simulink model "model"  (R2014a)
(part 6 of 6)

  bus4 : powerlib/Measurements/Load Flow Bus  LConnTagsString=a  ID=bus4  Vbase=10000  Vref=1  Vangle=0  VLF=1  angleLF=0
      settings: AttributesFormatString=|
      | %<ID>
      | %<Vbase>V
      | %<VLF>pu
      | %<angleLF>deg.
      | %<Name>
  bus40 : powerlib/Measurements/Load Flow Bus  LConnTagsString=a  ID=bus40  Vbase=10000  Vref=1  Vangle=0  VLF=1  angleLF=0
      settings: AttributesFormatString=|
      | %<ID>
      | %<Vbase>V
      | %<VLF>pu
      | %<angleLF>deg.
      | %<Name>
  bus41 : powerlib/Measurements/Load Flow Bus  LConnTagsString=a  ID=bus41  Vbase=10000  Vref=1  Vangle=0  VLF=1  angleLF=0
      settings: AttributesFormatString=|
      | %<ID>
      | %<Vbase>V
      | %<VLF>pu
      | %<angleLF>deg.
      | %<Name>
  bus42 : powerlib/Measurements/Load Flow Bus  LConnTagsString=a  ID=bus42  Vbase=10000  Vref=1  Vangle=0  VLF=1  angleLF=0
      settings: AttributesFormatString=|
      | %<ID>
      | %<Vbase>V
      | %<VLF>pu
      | %<angleLF>deg.
      | %<Name>
  bus43 : powerlib/Measurements/Load Flow Bus  LConnTagsString=a  ID=bus43  Vbase=10000  Vref=1  Vangle=0  VLF=1  angleLF=0
      settings: AttributesFormatString=|
      | %<ID>
      | %<Vbase>V
      | %<VLF>pu
      | %<angleLF>deg.
      | %<Name>
  bus44 : powerlib/Measurements/Load Flow Bus  LConnTagsString=a  ID=bus44  Vbase=10000  Vref=1  Vangle=0  VLF=1  angleLF=0
      settings: AttributesFormatString=|
      | %<ID>
      | %<Vbase>V
      | %<VLF>pu
      | %<angleLF>deg.
      | %<Name>
  bus45 : powerlib/Measurements/Load Flow Bus  LConnTagsString=a  ID=bus45  Vbase=10000  Vref=1  Vangle=0  VLF=1  angleLF=0
      settings: AttributesFormatString=|
      | %<ID>
      | %<Vbase>V
      | %<VLF>pu
      | %<angleLF>deg.
      | %<Name>
  bus46 : powerlib/Measurements/Load Flow Bus  LConnTagsString=a  ID=bus46  Vbase=10000  Vref=1  Vangle=0  VLF=1  angleLF=0
      settings: AttributesFormatString=|
      | %<ID>
      | %<Vbase>V
      | %<VLF>pu
      | %<angleLF>deg.
      | %<Name>
  bus47 : powerlib/Measurements/Load Flow Bus  LConnTagsString=a  ID=bus47  Vbase=10000  Vref=1  Vangle=0  VLF=1  angleLF=0
      settings: AttributesFormatString=|
      | %<ID>
      | %<Vbase>V
      | %<VLF>pu
      | %<angleLF>deg.
      | %<Name>
  bus48 : powerlib/Measurements/Load Flow Bus  LConnTagsString=a  ID=bus48  Vbase=10000  Vref=1  Vangle=0  VLF=1  angleLF=0
      settings: AttributesFormatString=|
      | %<ID>
      | %<Vbase>V
      | %<VLF>pu
      | %<angleLF>deg.
      | %<Name>
  bus49 : powerlib/Measurements/Load Flow Bus  LConnTagsString=a  ID=bus49  Vbase=10000  Vref=1  Vangle=0  VLF=1  angleLF=0
      settings: AttributesFormatString=|
      | %<ID>
      | %<Vbase>V
      | %<VLF>pu
      | %<angleLF>deg.
      | %<Name>
  bus5 : powerlib/Measurements/Load Flow Bus  LConnTagsString=a  ID=bus5  Vbase=10000  Vref=1  Vangle=0  VLF=1  angleLF=0
      settings: AttributesFormatString=|
      | %<ID>
      | %<Vbase>V
      | %<VLF>pu
      | %<angleLF>deg.
      | %<Name>
  bus50 : powerlib/Measurements/Load Flow Bus  LConnTagsString=a  ID=bus50  Vbase=10000  Vref=1  Vangle=0  VLF=1  angleLF=0
      settings: AttributesFormatString=|
      | %<ID>
      | %<Vbase>V
      | %<VLF>pu
      | %<angleLF>deg.
      | %<Name>
  bus51 : powerlib/Measurements/Load Flow Bus  LConnTagsString=a  ID=bus51  Vbase=10000  Vref=1  Vangle=0  VLF=1  angleLF=0
      settings: AttributesFormatString=|
      | %<ID>
      | %<Vbase>V
      | %<VLF>pu
      | %<angleLF>deg.
      | %<Name>
  bus52 : powerlib/Measurements/Load Flow Bus  LConnTagsString=a  ID=bus52  Vbase=10000  Vref=1  Vangle=0  VLF=1  angleLF=0
      settings: AttributesFormatString=|
      | %<ID>
      | %<Vbase>V
      | %<VLF>pu
      | %<angleLF>deg.
      | %<Name>
  bus53 : powerlib/Measurements/Load Flow Bus  LConnTagsString=a  ID=bus53  Vbase=10000  Vref=1  Vangle=0  VLF=1  angleLF=0
      settings: AttributesFormatString=|
      | %<ID>
      | %<Vbase>V
      | %<VLF>pu
      | %<angleLF>deg.
      | %<Name>
  bus54 : powerlib/Measurements/Load Flow Bus  LConnTagsString=a  ID=bus54  Vbase=10000  Vref=1  Vangle=0  VLF=1  angleLF=0
      settings: AttributesFormatString=|
      | %<ID>
      | %<Vbase>V
      | %<VLF>pu
      | %<angleLF>deg.
      | %<Name>
  bus55 : powerlib/Measurements/Load Flow Bus  LConnTagsString=a  ID=bus55  Vbase=10000  Vref=1  Vangle=0  VLF=1  angleLF=0
      settings: AttributesFormatString=|
      | %<ID>
      | %<Vbase>V
      | %<VLF>pu
      | %<angleLF>deg.
      | %<Name>
  bus56 : powerlib/Measurements/Load Flow Bus  LConnTagsString=a  ID=bus56  Vbase=10000  Vref=1  Vangle=0  VLF=1  angleLF=0
      settings: AttributesFormatString=|
      | %<ID>
      | %<Vbase>V
      | %<VLF>pu
      | %<angleLF>deg.
      | %<Name>
  bus57 : powerlib/Measurements/Load Flow Bus  LConnTagsString=a  ID=bus57  Vbase=10000  Vref=1  Vangle=0  VLF=1  angleLF=0
      settings: AttributesFormatString=|
      | %<ID>
      | %<Vbase>V
      | %<VLF>pu
      | %<angleLF>deg.
      | %<Name>
  bus58 : powerlib/Measurements/Load Flow Bus  LConnTagsString=a  ID=bus58  Vbase=10000  Vref=1  Vangle=0  VLF=1  angleLF=0
      settings: AttributesFormatString=|
      | %<ID>
      | %<Vbase>V
      | %<VLF>pu
      | %<angleLF>deg.
      | %<Name>
  bus59 : powerlib/Measurements/Load Flow Bus  LConnTagsString=a  ID=bus59  Vbase=10000  Vref=1  Vangle=0  VLF=1  angleLF=0
      settings: AttributesFormatString=|
      | %<ID>
      | %<Vbase>V
      | %<VLF>pu
      | %<angleLF>deg.
      | %<Name>
  bus6 : powerlib/Measurements/Load Flow Bus  LConnTagsString=a  ID=bus6  Vbase=10000  Vref=1  Vangle=0  VLF=1  angleLF=0
      settings: AttributesFormatString=|
      | %<ID>
      | %<Vbase>V
      | %<VLF>pu
      | %<angleLF>deg.
      | %<Name>
  bus60 : powerlib/Measurements/Load Flow Bus  LConnTagsString=a  ID=bus60  Vbase=10000  Vref=1  Vangle=0  VLF=1  angleLF=0
      settings: AttributesFormatString=|
      | %<ID>
      | %<Vbase>V
      | %<VLF>pu
      | %<angleLF>deg.
      | %<Name>
  bus61 : powerlib/Measurements/Load Flow Bus  LConnTagsString=a  ID=bus61  Vbase=10000  Vref=1  Vangle=0  VLF=1  angleLF=0
      settings: AttributesFormatString=|
      | %<ID>
      | %<Vbase>V
      | %<VLF>pu
      | %<angleLF>deg.
      | %<Name>
  bus62 : powerlib/Measurements/Load Flow Bus  LConnTagsString=a  ID=bus62  Vbase=10000  Vref=1  Vangle=0  VLF=1  angleLF=0
      settings: AttributesFormatString=|
      | %<ID>
      | %<Vbase>V
      | %<VLF>pu
      | %<angleLF>deg.
      | %<Name>
  bus63 : powerlib/Measurements/Load Flow Bus  LConnTagsString=a  ID=bus63  Vbase=10000  Vref=1  Vangle=0  VLF=1  angleLF=0
      settings: AttributesFormatString=|
      | %<ID>
      | %<Vbase>V
      | %<VLF>pu
      | %<angleLF>deg.
      | %<Name>
  bus64 : powerlib/Measurements/Load Flow Bus  LConnTagsString=a  ID=bus64  Vbase=10000  Vref=1  Vangle=0  VLF=1  angleLF=0
      settings: AttributesFormatString=|
      | %<ID>
      | %<Vbase>V
      | %<VLF>pu
      | %<angleLF>deg.
      | %<Name>
  bus65 : powerlib/Measurements/Load Flow Bus  LConnTagsString=a  ID=bus65  Vbase=10000  Vref=1  Vangle=0  VLF=1  angleLF=0
      settings: AttributesFormatString=|
      | %<ID>
      | %<Vbase>V
      | %<VLF>pu
      | %<angleLF>deg.
      | %<Name>
  bus66 : powerlib/Measurements/Load Flow Bus  LConnTagsString=a  ID=bus66  Vbase=10000  Vref=1  Vangle=0  VLF=1  angleLF=0
      settings: AttributesFormatString=|
      | %<ID>
      | %<Vbase>V
      | %<VLF>pu
      | %<angleLF>deg.
      | %<Name>
  bus67 : powerlib/Measurements/Load Flow Bus  LConnTagsString=a  ID=bus67  Vbase=10000  Vref=1  Vangle=0  VLF=1  angleLF=0
      settings: AttributesFormatString=|
      | %<ID>
      | %<Vbase>V
      | %<VLF>pu
      | %<angleLF>deg.
      | %<Name>
  bus68 : powerlib/Measurements/Load Flow Bus  LConnTagsString=a  ID=bus68  Vbase=10000  Vref=1  Vangle=0  VLF=1  angleLF=0
      settings: AttributesFormatString=|
      | %<ID>
      | %<Vbase>V
      | %<VLF>pu
      | %<angleLF>deg.
      | %<Name>
  bus69 : powerlib/Measurements/Load Flow Bus  LConnTagsString=a  ID=bus69  Vbase=10000  Vref=1  Vangle=0  VLF=1  angleLF=0
      settings: AttributesFormatString=|
      | %<ID>
      | %<Vbase>V
      | %<VLF>pu
      | %<angleLF>deg.
      | %<Name>
  bus7 : powerlib/Measurements/Load Flow Bus  LConnTagsString=a  ID=bus7  Vbase=10000  Vref=1  Vangle=0  VLF=1  angleLF=0
      settings: AttributesFormatString=|
      | %<ID>
      | %<Vbase>V
      | %<VLF>pu
      | %<angleLF>deg.
      | %<Name>
  bus70 : powerlib/Measurements/Load Flow Bus  LConnTagsString=a  ID=bus70  Vbase=10000  Vref=1  Vangle=0  VLF=1  angleLF=0
      settings: AttributesFormatString=|
      | %<ID>
      | %<Vbase>V
      | %<VLF>pu
      | %<angleLF>deg.
      | %<Name>
  bus71 : powerlib/Measurements/Load Flow Bus  LConnTagsString=a  ID=bus71  Vbase=10000  Vref=1  Vangle=0  VLF=1  angleLF=0
      settings: AttributesFormatString=|
      | %<ID>
      | %<Vbase>V
      | %<VLF>pu
      | %<angleLF>deg.
      | %<Name>
  bus72 : powerlib/Measurements/Load Flow Bus  LConnTagsString=a  ID=bus72  Vbase=10000  Vref=1  Vangle=0  VLF=1  angleLF=0
      settings: AttributesFormatString=|
      | %<ID>
      | %<Vbase>V
      | %<VLF>pu
      | %<angleLF>deg.
      | %<Name>
  bus73 : powerlib/Measurements/Load Flow Bus  LConnTagsString=a  ID=bus73  Vbase=10000  Vref=1  Vangle=0  VLF=1  angleLF=0
      settings: AttributesFormatString=|
      | %<ID>
      | %<Vbase>V
      | %<VLF>pu
      | %<angleLF>deg.
      | %<Name>
  bus74 : powerlib/Measurements/Load Flow Bus  LConnTagsString=a  ID=bus74  Vbase=10000  Vref=1  Vangle=0  VLF=1  angleLF=0
      settings: AttributesFormatString=|
      | %<ID>
      | %<Vbase>V
      | %<VLF>pu
      | %<angleLF>deg.
      | %<Name>
  bus75 : powerlib/Measurements/Load Flow Bus  LConnTagsString=a  ID=bus75  Vbase=33000  Vref=1  Vangle=0  VLF=1  angleLF=0
      settings: AttributesFormatString=|
      | %<ID>
      | %<Vbase>V
      | %<VLF>pu
      | %<angleLF>deg.
      | %<Name>
  bus76 : powerlib/Measurements/Load Flow Bus  LConnTagsString=a  ID=bus76  Vbase=33000  Vref=1  Vangle=0  VLF=1  angleLF=0
      settings: AttributesFormatString=|
      | %<ID>
      | %<Vbase>V
      | %<VLF>pu
      | %<angleLF>deg.
      | %<Name>
  bus77 : powerlib/Measurements/Load Flow Bus  LConnTagsString=a  ID=bus77  Vbase=33000  Vref=1  Vangle=0  VLF=1  angleLF=0
      settings: AttributesFormatString=|
      | %<ID>
      | %<Vbase>V
      | %<VLF>pu
      | %<angleLF>deg.
      | %<Name>
  bus78 : powerlib/Measurements/Load Flow Bus  LConnTagsString=a  ID=bus78  Vbase=33000  Vref=1  Vangle=0  VLF=1  angleLF=0
      settings: AttributesFormatString=|
      | %<ID>
      | %<Vbase>V
      | %<VLF>pu
      | %<angleLF>deg.
      | %<Name>
  bus79 : powerlib/Measurements/Load Flow Bus  LConnTagsString=a  ID=bus79  Vbase=33000  Vref=1  Vangle=0  VLF=1  angleLF=0
      settings: AttributesFormatString=|
      | %<ID>
      | %<Vbase>V
      | %<VLF>pu
      | %<angleLF>deg.
      | %<Name>
  bus8 : powerlib/Measurements/Load Flow Bus  LConnTagsString=a  ID=bus8  Vbase=10000  Vref=1  Vangle=0  VLF=1  angleLF=0
      settings: AttributesFormatString=|
      | %<ID>
      | %<Vbase>V
      | %<VLF>pu
      | %<angleLF>deg.
      | %<Name>
  bus80 : powerlib/Measurements/Load Flow Bus  LConnTagsString=a  ID=bus80  Vbase=33000  Vref=1  Vangle=0  VLF=1  angleLF=0
      settings: AttributesFormatString=|
      | %<ID>
      | %<Vbase>V
      | %<VLF>pu
      | %<angleLF>deg.
      | %<Name>
  bus81 : powerlib/Measurements/Load Flow Bus  LConnTagsString=a  ID=bus81  Vbase=33000  Vref=1  Vangle=0  VLF=1  angleLF=0
      settings: AttributesFormatString=|
      | %<ID>
      | %<Vbase>V
      | %<VLF>pu
      | %<angleLF>deg.
      | %<Name>
  bus82 : powerlib/Measurements/Load Flow Bus  LConnTagsString=a  ID=bus82  Vbase=33000  Vref=1  Vangle=0  VLF=1  angleLF=0
      settings: AttributesFormatString=|
      | %<ID>
      | %<Vbase>V
      | %<VLF>pu
      | %<angleLF>deg.
      | %<Name>
  bus83 : powerlib/Measurements/Load Flow Bus  LConnTagsString=a  ID=bus83  Vbase=33000  Vref=1  Vangle=0  VLF=1  angleLF=0
      settings: AttributesFormatString=|
      | %<ID>
      | %<Vbase>V
      | %<VLF>pu
      | %<angleLF>deg.
      | %<Name>
  bus84 : powerlib/Measurements/Load Flow Bus  LConnTagsString=a  ID=bus84  Vbase=33000  Vref=1  Vangle=0  VLF=1  angleLF=0
      settings: AttributesFormatString=|
      | %<ID>
      | %<Vbase>V
      | %<VLF>pu
      | %<angleLF>deg.
      | %<Name>
  bus85 : powerlib/Measurements/Load Flow Bus  LConnTagsString=a  ID=bus85  Vbase=33000  Vref=1  Vangle=0  VLF=1  angleLF=0
      settings: AttributesFormatString=|
      | %<ID>
      | %<Vbase>V
      | %<VLF>pu
      | %<angleLF>deg.
      | %<Name>
  bus86 : powerlib/Measurements/Load Flow Bus  LConnTagsString=a  ID=bus86  Vbase=33000  Vref=1  Vangle=0  VLF=1  angleLF=0
      settings: AttributesFormatString=|
      | %<ID>
      | %<Vbase>V
      | %<VLF>pu
      | %<angleLF>deg.
      | %<Name>
  bus87 : powerlib/Measurements/Load Flow Bus  LConnTagsString=a  ID=bus87  Vbase=33000  Vref=1  Vangle=0  VLF=1  angleLF=0
      settings: AttributesFormatString=|
      | %<ID>
      | %<Vbase>V
      | %<VLF>pu
      | %<angleLF>deg.
      | %<Name>
  bus88 : powerlib/Measurements/Load Flow Bus  LConnTagsString=a  ID=bus88  Vbase=33000  Vref=1  Vangle=0  VLF=1  angleLF=0
      settings: AttributesFormatString=|
      | %<ID>
      | %<Vbase>V
      | %<VLF>pu
      | %<angleLF>deg.
      | %<Name>
  bus89 : powerlib/Measurements/Load Flow Bus  LConnTagsString=a  ID=bus89  Vbase=33000  Vref=1  Vangle=0  VLF=1  angleLF=0
      settings: AttributesFormatString=|
      | %<ID>
      | %<Vbase>V
      | %<VLF>pu
      | %<angleLF>deg.
      | %<Name>
  bus9 : powerlib/Measurements/Load Flow Bus  LConnTagsString=a  ID=bus9  Vbase=10000  Vref=1  Vangle=0  VLF=1  angleLF=0
      settings: AttributesFormatString=|
      | %<ID>
      | %<Vbase>V
      | %<VLF>pu
      | %<angleLF>deg.
      | %<Name>
  bus90 : powerlib/Measurements/Load Flow Bus  LConnTagsString=a  ID=bus90  Vbase=33000  Vref=1  Vangle=0  VLF=1  angleLF=0
      settings: AttributesFormatString=|
      | %<ID>
      | %<Vbase>V
      | %<VLF>pu
      | %<angleLF>deg.
      | %<Name>
  bus91 : powerlib/Measurements/Load Flow Bus  LConnTagsString=a  ID=bus91  Vbase=33000  Vref=1  Vangle=0  VLF=1  angleLF=0
      settings: AttributesFormatString=|
      | %<ID>
      | %<Vbase>V
      | %<VLF>pu
      | %<angleLF>deg.
      | %<Name>
  bus92 : powerlib/Measurements/Load Flow Bus  LConnTagsString=a  ID=bus92  Vbase=33000  Vref=1  Vangle=0  VLF=1  angleLF=0
      settings: AttributesFormatString=|
      | %<ID>
      | %<Vbase>V
      | %<VLF>pu
      | %<angleLF>deg.
      | %<Name>
  bus93 : powerlib/Measurements/Load Flow Bus  LConnTagsString=a  ID=bus93  Vbase=33000  Vref=1  Vangle=0  VLF=1  angleLF=0
      settings: AttributesFormatString=|
      | %<ID>
      | %<Vbase>V
      | %<VLF>pu
      | %<angleLF>deg.
      | %<Name>
  bus94 : powerlib/Measurements/Load Flow Bus  LConnTagsString=a  ID=bus94  Vbase=33000  Vref=1  Vangle=0  VLF=1  angleLF=0
      settings: AttributesFormatString=|
      | %<ID>
      | %<Vbase>V
      | %<VLF>pu
      | %<angleLF>deg.
      | %<Name>
  bus95 : powerlib/Measurements/Load Flow Bus  LConnTagsString=a  ID=bus95  Vbase=33000  Vref=1  Vangle=0  VLF=1  angleLF=0
      settings: AttributesFormatString=|
      | %<ID>
      | %<Vbase>V
      | %<VLF>pu
      | %<angleLF>deg.
      | %<Name>
  bus96 : powerlib/Measurements/Load Flow Bus  LConnTagsString=a  ID=bus96  Vbase=33000  Vref=1  Vangle=0  VLF=1  angleLF=0
      settings: AttributesFormatString=|
      | %<ID>
      | %<Vbase>V
      | %<VLF>pu
      | %<angleLF>deg.
      | %<Name>
  bus97 : powerlib/Measurements/Load Flow Bus  LConnTagsString=a  ID=bus97  Vbase=33000  Vref=1  Vangle=0  VLF=1  angleLF=0
      settings: AttributesFormatString=|
      | %<ID>
      | %<Vbase>V
      | %<VLF>pu
      | %<angleLF>deg.
      | %<Name>
  bus98 : powerlib/Measurements/Load Flow Bus  LConnTagsString=a  ID=bus98  Vbase=33000  Vref=1  Vangle=0  VLF=1  angleLF=0
      settings: AttributesFormatString=|
      | %<ID>
      | %<Vbase>V
      | %<VLF>pu
      | %<angleLF>deg.
      | %<Name>
  bus99 : powerlib/Measurements/Load Flow Bus  LConnTagsString=a  ID=bus99  Vbase=35000  Vref=1  Vangle=0  VLF=1  angleLF=0
      settings: AttributesFormatString=|
      | %<ID>
      | %<Vbase>V
      | %<VLF>pu
      | %<angleLF>deg.
      | %<Name>
  powergui : powerlib/powergui  Priority=1  SimulationMode=Continuous  SolverType=Tustin  SampleTime=50e-6  frequency=60  SPID=off  DisableSnubberDevices=off  DisableRonSwitches=off  DisableVfSwitches=off  SwTol=0  Interpol=off  DisplayEquations=off  Ts=0  methode=off  frequencyindice=60  Pbase=100e6  ErrMax=1e-4  Iterations=50  UnitsV=kV  UnitsW=MW  FunctionMessages=off  echomessages=off  HookPort=off  EnableUseOfTLC=off  x0status=blocks  RestoreLinks=warning  ResistiveCurrentMeasurement=off  Frange=[0:2:500]  Ylog=off  Xlog=on  ShowGrid=off  save=off  variable=ZData  structure=0  ZoomFFT=off  StartTime=0.0  cycles=1  DisplayStyle=1  fundamental=60  FreqAxis=off  MaxFrequency=1000  frequencyindicesteady=1  RmsSteady=1  display=off
  Ötztal___Zirl_CN_147563007_110000_CN_100404264_110000 : powerlib/Elements/Distributed Parameters Line  Phases=3  Frequency=60  Resistance=[0.01273 0.3864]  Inductance="[0.9337e-3  4.1264e-3]"  Capacitance=[12.74e-9 7.751e-9]  Length=100  x1=[0 0 0 0; 0.0001244 0 0 0; 0.0002488 0 0 0; 0.0003733 0 0 0; 0.0004977 0 0 0; 0.0006221 0 0 0]  x2=[0 0 0 0; 0.0001244 0 0 0; 0.0002488 0 0 0; 0.0003733 0 0 0; 0.0004977 0 0 0; 0.0006221 0 0 0]  x3=[0 0 0 0; 0.0001244 0 0 0; 0.0002488 0 0 0; 0.0003733 0 0 0; 0.0004977 0 0 0; 0.0006221 0 0 0]  x4=[0 0 0 0; 0.0001244 0 0 0; 0.0002488 0 0 0; 0.0003733 0 0 0; 0.0004977 0 0 0; 0.0006221 0 0 0]  x5=0  V1=ones(3,3)  V2=ones(3,3)  I1=ones(3,3)  I2=ones(3,3)  nHarmo=1  Measurements=None
  connections:
  _CN_46584322_10000_CN_41794316_10000/LConn1 -- T_46584322__/RConn1 -- _CN_46584322_10000_CN_48374400_10000/LConn1 -- L_46584322/LConn1
  _CN_46584322_10000_CN_41794316_10000/LConn2 -- T_46584322__/RConn2 -- _CN_46584322_10000_CN_48374400_10000/LConn2 -- L_46584322/LConn2
  _CN_46584322_10000_CN_41794316_10000/LConn3 -- T_46584322__/RConn3 -- _CN_46584322_10000_CN_48374400_10000/LConn3 -- L_46584322/LConn3 -- bus1/LConn1
  _CN_46584322_10000_CN_41794316_10000/RConn1 -- T_41794316__/RConn1 -- _CN_92224085_10000_CN_41794316_10000/LConn1 -- _CN_46587556_10000_CN_41794316_10000/LConn1 -- _CN_117198289_10000_CN_41794316_10000/LConn1 -- L_41794316/LConn1
  _CN_46584322_10000_CN_41794316_10000/RConn2 -- T_41794316__/RConn2 -- _CN_92224085_10000_CN_41794316_10000/LConn2 -- _CN_46587556_10000_CN_41794316_10000/LConn2 -- _CN_117198289_10000_CN_41794316_10000/LConn2 -- L_41794316/LConn2
  _CN_46584322_10000_CN_41794316_10000/RConn3 -- T_41794316__/RConn3 -- _CN_92224085_10000_CN_41794316_10000/LConn3 -- _CN_46587556_10000_CN_41794316_10000/LConn3 -- _CN_117198289_10000_CN_41794316_10000/LConn3 -- L_41794316/LConn3 -- bus2/LConn1
  T_48374400__/LConn1 -- _CN_46584322_10000_CN_48374400_10000/RConn1
  T_48374400__/LConn2 -- _CN_46584322_10000_CN_48374400_10000/RConn2
  _CN_46584322_10000_CN_48374400_10000/RConn3 -- T_48374400__/LConn3 -- bus3/LConn1
  _CN_85643780_10000_CN_83892667_10000/LConn1 -- T_85643780__/LConn1 -- _CN_85643780_10000_CN_100419275_10000/LConn1 -- _CN_85643780_10000_CN_67678755_10000/LConn1
  _CN_85643780_10000_CN_83892667_10000/LConn2 -- T_85643780__/LConn2 -- _CN_85643780_10000_CN_100419275_10000/LConn2 -- _CN_85643780_10000_CN_67678755_10000/LConn2
  _CN_85643780_10000_CN_83892667_10000/LConn3 -- T_85643780__/LConn3 -- _CN_85643780_10000_CN_100419275_10000/LConn3 -- _CN_85643780_10000_CN_67678755_10000/LConn3 -- bus4/LConn1
  T_83892667__/LConn1 -- _CN_85643780_10000_CN_83892667_10000/RConn1
  T_83892667__/LConn2 -- _CN_85643780_10000_CN_83892667_10000/RConn2
  _CN_85643780_10000_CN_83892667_10000/RConn3 -- T_83892667__/LConn3 -- bus5/LConn1
  T_100419275__/LConn1 -- _CN_85643780_10000_CN_100419275_10000/RConn1
  T_100419275__/LConn2 -- _CN_85643780_10000_CN_100419275_10000/RConn2
  _CN_85643780_10000_CN_100419275_10000/RConn3 -- T_100419275__/LConn3 -- bus6/LConn1
  T_67678755__/LConn1 -- _CN_85643780_10000_CN_67678755_10000/RConn1
  T_67678755__/LConn2 -- _CN_85643780_10000_CN_67678755_10000/RConn2
  _CN_85643780_10000_CN_67678755_10000/RConn3 -- T_67678755__/LConn3 -- bus7/LConn1
  T_93799430__/LConn1 -- _CN_93799430_10000_CN_85256767_10000/LConn1
  T_93799430__/LConn2 -- _CN_93799430_10000_CN_85256767_10000/LConn2
  _CN_93799430_10000_CN_85256767_10000/LConn3 -- T_93799430__/LConn3 -- bus8/LConn1
  _CN_93799430_10000_CN_85256767_10000/RConn1 -- T_85256767__/RConn1 -- L_85256767/LConn1
  _CN_93799430_10000_CN_85256767_10000/RConn2 -- T_85256767__/RConn2 -- L_85256767/LConn2
  _CN_93799430_10000_CN_85256767_10000/RConn3 -- T_85256767__/RConn3 -- L_85256767/LConn3 -- bus9/LConn1
  _CN_43176990_10000_CN_43201849_10000/LConn1 -- T_43176990__/RConn1 -- L_43176990/LConn1
  _CN_43176990_10000_CN_43201849_10000/LConn2 -- T_43176990__/RConn2 -- L_43176990/LConn2
  _CN_43176990_10000_CN_43201849_10000/LConn3 -- T_43176990__/RConn3 -- L_43176990/LConn3 -- bus10/LConn1
  _CN_43176990_10000_CN_43201849_10000/RConn1 -- T_43201849__подстанция_Южная/RConn1 -- L_43201849/LConn1
  _CN_43176990_10000_CN_43201849_10000/RConn2 -- T_43201849__подстанция_Южная/RConn2 -- L_43201849/LConn2
  _CN_43176990_10000_CN_43201849_10000/RConn3 -- T_43201849__подстанция_Южная/RConn3 -- L_43201849/LConn3 -- bus11/LConn1
  "T_33533471__PDC_11_\"Zorile\""/LConn1 -- _CN_33533471_10000_CN_33187294_10000/LConn1
  "T_33533471__PDC_11_\"Zorile\""/LConn2 -- _CN_33533471_10000_CN_33187294_10000/LConn2
  _CN_33533471_10000_CN_33187294_10000/LConn3 -- "T_33533471__PDC_11_\"Zorile\""/LConn3 -- bus12/LConn1
  _CN_33533471_10000_CN_33187294_10000/RConn1 -- "T_33187294_110000_PDC_1_\"Sculeni\""/LConn1 -- _CN_33187294_10000_CN_33187300_10000/LConn1
  _CN_33533471_10000_CN_33187294_10000/RConn2 -- "T_33187294_110000_PDC_1_\"Sculeni\""/LConn2 -- _CN_33187294_10000_CN_33187300_10000/LConn2
  _CN_33533471_10000_CN_33187294_10000/RConn3 -- "T_33187294_110000_PDC_1_\"Sculeni\""/LConn3 -- _CN_33187294_10000_CN_33187300_10000/LConn3 -- bus13/LConn1
  T_104961071__/LConn1 -- _CN_104961071_10000_CN_104845142_10000/LConn1
  T_104961071__/LConn2 -- _CN_104961071_10000_CN_104845142_10000/LConn2
  _CN_104961071_10000_CN_104845142_10000/LConn3 -- T_104961071__/LConn3 -- bus14/LConn1
  T_104845142__/LConn1 -- _CN_104961071_10000_CN_104845142_10000/RConn1
  T_104845142__/LConn2 -- _CN_104961071_10000_CN_104845142_10000/RConn2
  _CN_104961071_10000_CN_104845142_10000/RConn3 -- T_104845142__/LConn3 -- bus15/LConn1
  T_43177004__/LConn1 -- _CN_43177004_10000_CN_43177007_10000/LConn1
  T_43177004__/LConn2 -- _CN_43177004_10000_CN_43177007_10000/LConn2
  _CN_43177004_10000_CN_43177007_10000/LConn3 -- T_43177004__/LConn3 -- bus16/LConn1
  T_43177007__/LConn1 -- _CN_43177004_10000_CN_43177007_10000/RConn1
  T_43177007__/LConn2 -- _CN_43177004_10000_CN_43177007_10000/RConn2
  _CN_43177004_10000_CN_43177007_10000/RConn3 -- T_43177007__/LConn3 -- bus17/LConn1
  T_49437741__/LConn1 -- _CN_49437741_10000_CN_49516591_10000/LConn1
  T_49437741__/LConn2 -- _CN_49437741_10000_CN_49516591_10000/LConn2
  _CN_49437741_10000_CN_49516591_10000/LConn3 -- T_49437741__/LConn3 -- bus18/LConn1
  T_49516591__/LConn1 -- _CN_49437741_10000_CN_49516591_10000/RConn1
  T_49516591__/LConn2 -- _CN_49437741_10000_CN_49516591_10000/RConn2
  _CN_49437741_10000_CN_49516591_10000/RConn3 -- T_49516591__/LConn3 -- bus19/LConn1
  _CN_89214520_10000_CN_40426094_10000/LConn1 -- T_89214520__/LConn1 -- _CN_89214520_10000_CN_108303571_10000/LConn1
  _CN_89214520_10000_CN_40426094_10000/LConn2 -- T_89214520__/LConn2 -- _CN_89214520_10000_CN_108303571_10000/LConn2
  _CN_89214520_10000_CN_40426094_10000/LConn3 -- T_89214520__/LConn3 -- _CN_89214520_10000_CN_108303571_10000/LConn3 -- bus20/LConn1
  _CN_89214520_10000_CN_40426094_10000/RConn1 -- T_40426094__/RConn1 -- L_40426094/LConn1
  _CN_89214520_10000_CN_40426094_10000/RConn2 -- T_40426094__/RConn2 -- L_40426094/LConn2
  _CN_89214520_10000_CN_40426094_10000/RConn3 -- T_40426094__/RConn3 -- L_40426094/LConn3 -- bus21/LConn1
  T_108303571__/LConn1 -- _CN_89214520_10000_CN_108303571_10000/RConn1
  T_108303571__/LConn2 -- _CN_89214520_10000_CN_108303571_10000/RConn2
  _CN_89214520_10000_CN_108303571_10000/RConn3 -- T_108303571__/LConn3 -- bus22/LConn1
  T_92839994__/LConn1 -- _CN_92839994_10000_CN_51199909_10000/LConn1
  T_92839994__/LConn2 -- _CN_92839994_10000_CN_51199909_10000/LConn2
  _CN_92839994_10000_CN_51199909_10000/LConn3 -- T_92839994__/LConn3 -- bus23/LConn1
  T_51199909__/LConn1 -- _CN_92839994_10000_CN_51199909_10000/RConn1
  T_51199909__/LConn2 -- _CN_92839994_10000_CN_51199909_10000/RConn2
  _CN_92839994_10000_CN_51199909_10000/RConn3 -- T_51199909__/LConn3 -- bus24/LConn1
  T_67678785__/LConn1 -- _CN_67678785_10000_CN_53211725_10000/LConn1
  T_67678785__/LConn2 -- _CN_67678785_10000_CN_53211725_10000/LConn2
  _CN_67678785_10000_CN_53211725_10000/LConn3 -- T_67678785__/LConn3 -- bus25/LConn1
  T_53211725__/LConn1 -- _CN_67678785_10000_CN_53211725_10000/RConn1
  T_53211725__/LConn2 -- _CN_67678785_10000_CN_53211725_10000/RConn2
  _CN_67678785_10000_CN_53211725_10000/RConn3 -- T_53211725__/LConn3 -- bus26/LConn1
  "T_38634061__PDC_35_\"Combinatul_de_Carton\""/LConn1 -- _CN_38634061_10000_CN_48274938_10000/LConn1
  "T_38634061__PDC_35_\"Combinatul_de_Carton\""/LConn2 -- _CN_38634061_10000_CN_48274938_10000/LConn2
  _CN_38634061_10000_CN_48274938_10000/LConn3 -- "T_38634061__PDC_35_\"Combinatul_de_Carton\""/LConn3 -- bus27/LConn1
  T_48274938__/LConn1 -- _CN_38634061_10000_CN_48274938_10000/RConn1
  T_48274938__/LConn2 -- _CN_38634061_10000_CN_48274938_10000/RConn2
  _CN_38634061_10000_CN_48274938_10000/RConn3 -- T_48274938__/LConn3 -- bus28/LConn1
  _CN_96687188_10000_CN_44046948_10000/LConn1 -- T_96687188__/LConn1 -- _CN_96687188_10000_CN_96689384_10000/LConn1
  _CN_96687188_10000_CN_44046948_10000/LConn2 -- T_96687188__/LConn2 -- _CN_96687188_10000_CN_96689384_10000/LConn2
  _CN_96687188_10000_CN_44046948_10000/LConn3 -- T_96687188__/LConn3 -- _CN_96687188_10000_CN_96689384_10000/LConn3 -- bus29/LConn1
  T_44046948__/LConn1 -- _CN_96687188_10000_CN_44046948_10000/RConn1
  T_44046948__/LConn2 -- _CN_96687188_10000_CN_44046948_10000/RConn2
  _CN_96687188_10000_CN_44046948_10000/RConn3 -- T_44046948__/LConn3 -- bus30/LConn1
  T_96689384__/LConn1 -- _CN_96687188_10000_CN_96689384_10000/RConn1
  T_96689384__/LConn2 -- _CN_96687188_10000_CN_96689384_10000/RConn2
  _CN_96687188_10000_CN_96689384_10000/RConn3 -- T_96689384__/LConn3 -- bus31/LConn1
  _CN_92224085_10000_CN_92224738_10000/LConn1 -- T_92224085__/RConn1 -- _CN_92224085_10000_CN_41794316_10000/RConn1 -- L_92224085/LConn1
  _CN_92224085_10000_CN_92224738_10000/LConn2 -- T_92224085__/RConn2 -- _CN_92224085_10000_CN_41794316_10000/RConn2 -- L_92224085/LConn2
  _CN_92224085_10000_CN_92224738_10000/LConn3 -- T_92224085__/RConn3 -- _CN_92224085_10000_CN_41794316_10000/RConn3 -- L_92224085/LConn3 -- bus32/LConn1
  T_92224738__/LConn1 -- _CN_92224085_10000_CN_92224738_10000/RConn1
  T_92224738__/LConn2 -- _CN_92224085_10000_CN_92224738_10000/RConn2
  _CN_92224085_10000_CN_92224738_10000/RConn3 -- T_92224738__/LConn3 -- bus33/LConn1
  T_93805661__/LConn1 -- _CN_93805661_10000_CN_59611290_10000/LConn1
  T_93805661__/LConn2 -- _CN_93805661_10000_CN_59611290_10000/LConn2
  _CN_93805661_10000_CN_59611290_10000/LConn3 -- T_93805661__/LConn3 -- bus34/LConn1
  T_59611290__/LConn1 -- _CN_93805661_10000_CN_59611290_10000/RConn1
  T_59611290__/LConn2 -- _CN_93805661_10000_CN_59611290_10000/RConn2
  _CN_93805661_10000_CN_59611290_10000/RConn3 -- T_59611290__/LConn3 -- bus35/LConn1
  T_33533030__PDC_13_„Albișoara”/LConn1 -- _CN_33533030_10000_CN_25799789_10000/LConn1
  T_33533030__PDC_13_„Albișoara”/LConn2 -- _CN_33533030_10000_CN_25799789_10000/LConn2
  _CN_33533030_10000_CN_25799789_10000/LConn3 -- T_33533030__PDC_13_„Albișoara”/LConn3 -- bus36/LConn1
  G_25799789_CET_2/RConn1 -- _CN_33533030_10000_CN_25799789_10000/RConn1
  G_25799789_CET_2/RConn2 -- _CN_33533030_10000_CN_25799789_10000/RConn2
  _CN_33533030_10000_CN_25799789_10000/RConn3 -- G_25799789_CET_2/RConn3 -- bus37/LConn1
  "T_33075316__PDC_12_\"Malina_Noua\""/LConn1 -- _CN_33075316_10000_CN_27835275_10000/LConn1
  "T_33075316__PDC_12_\"Malina_Noua\""/LConn2 -- _CN_33075316_10000_CN_27835275_10000/LConn2
  _CN_33075316_10000_CN_27835275_10000/LConn3 -- "T_33075316__PDC_12_\"Malina_Noua\""/LConn3 -- bus38/LConn1
  _CN_33075316_10000_CN_27835275_10000/RConn1 -- "T_27835275__PDC_\"Chișinău_Sud\""/RConn4 -- L_27835275/LConn1
  _CN_33075316_10000_CN_27835275_10000/RConn2 -- "T_27835275__PDC_\"Chișinău_Sud\""/RConn5 -- L_27835275/LConn2
  _CN_33075316_10000_CN_27835275_10000/RConn3 -- "T_27835275__PDC_\"Chișinău_Sud\""/RConn6 -- L_27835275/LConn3 -- bus39/LConn1
  T_106050843__/LConn1 -- _CN_106050843_10000_CN_106050849_10000/LConn1
  T_106050843__/LConn2 -- _CN_106050843_10000_CN_106050849_10000/LConn2
  _CN_106050843_10000_CN_106050849_10000/LConn3 -- T_106050843__/LConn3 -- bus40/LConn1
  T_106050849__/LConn1 -- _CN_106050843_10000_CN_106050849_10000/RConn1
  T_106050849__/LConn2 -- _CN_106050843_10000_CN_106050849_10000/RConn2
  _CN_106050843_10000_CN_106050849_10000/RConn3 -- T_106050849__/LConn3 -- bus41/LConn1
  _CN_46587556_10000_CN_36056921_10000/LConn1 -- T_46587556__/LConn1 -- _CN_46587556_10000_CN_50287787_10000/LConn1 -- _CN_46587556_10000_CN_50287791_10000/LConn1 -- _CN_46587556_10000_CN_41794316_10000/RConn1
  _CN_46587556_10000_CN_36056921_10000/LConn2 -- T_46587556__/LConn2 -- _CN_46587556_10000_CN_50287787_10000/LConn2 -- _CN_46587556_10000_CN_50287791_10000/LConn2 -- _CN_46587556_10000_CN_41794316_10000/RConn2
  _CN_46587556_10000_CN_36056921_10000/LConn3 -- T_46587556__/LConn3 -- _CN_46587556_10000_CN_50287787_10000/LConn3 -- _CN_46587556_10000_CN_50287791_10000/LConn3 -- _CN_46587556_10000_CN_41794316_10000/RConn3 -- bus42/LConn1
  T_36056921__/LConn1 -- _CN_46587556_10000_CN_36056921_10000/RConn1
  T_36056921__/LConn2 -- _CN_46587556_10000_CN_36056921_10000/RConn2
  _CN_46587556_10000_CN_36056921_10000/RConn3 -- T_36056921__/LConn3 -- bus43/LConn1
  T_50287787__/LConn1 -- _CN_46587556_10000_CN_50287787_10000/RConn1
  T_50287787__/LConn2 -- _CN_46587556_10000_CN_50287787_10000/RConn2
  _CN_46587556_10000_CN_50287787_10000/RConn3 -- T_50287787__/LConn3 -- bus44/LConn1
  T_50287791__/LConn1 -- _CN_46587556_10000_CN_50287791_10000/RConn1
  T_50287791__/LConn2 -- _CN_46587556_10000_CN_50287791_10000/RConn2
  _CN_46587556_10000_CN_50287791_10000/RConn3 -- T_50287791__/LConn3 -- bus45/LConn1
  _CN_96335020_10000_CN_96335030_10000/LConn1 -- T_96335020__/LConn1 -- _CN_96335020_10000_CN_96335034_10000/LConn1
  _CN_96335020_10000_CN_96335030_10000/LConn2 -- T_96335020__/LConn2 -- _CN_96335020_10000_CN_96335034_10000/LConn2
  _CN_96335020_10000_CN_96335030_10000/LConn3 -- T_96335020__/LConn3 -- _CN_96335020_10000_CN_96335034_10000/LConn3 -- bus46/LConn1
  T_96335030__/LConn1 -- _CN_96335020_10000_CN_96335030_10000/RConn1
  T_96335030__/LConn2 -- _CN_96335020_10000_CN_96335030_10000/RConn2
  _CN_96335020_10000_CN_96335030_10000/RConn3 -- T_96335030__/LConn3 -- bus47/LConn1
  T_96335034__/LConn1 -- _CN_96335020_10000_CN_96335034_10000/RConn1
  T_96335034__/LConn2 -- _CN_96335020_10000_CN_96335034_10000/RConn2
  _CN_96335020_10000_CN_96335034_10000/RConn3 -- T_96335034__/LConn3 -- bus48/LConn1
  T_92235449__/LConn1 -- _CN_92235449_10000_CN_95423979_10000/LConn1
  T_92235449__/LConn2 -- _CN_92235449_10000_CN_95423979_10000/LConn2
  _CN_92235449_10000_CN_95423979_10000/LConn3 -- T_92235449__/LConn3 -- bus49/LConn1
  _CN_92235449_10000_CN_95423979_10000/RConn1 -- T_95423979__/LConn1 -- _CN_95423979_10000_CN_92385772_10000/LConn1
  _CN_92235449_10000_CN_95423979_10000/RConn2 -- T_95423979__/LConn2 -- _CN_95423979_10000_CN_92385772_10000/LConn2
  _CN_92235449_10000_CN_95423979_10000/RConn3 -- T_95423979__/LConn3 -- _CN_95423979_10000_CN_92385772_10000/LConn3 -- bus50/LConn1
  T_86014138__/LConn1 -- _CN_86014138_10000_CN_45274398_10000/LConn1
  T_86014138__/LConn2 -- _CN_86014138_10000_CN_45274398_10000/LConn2
  _CN_86014138_10000_CN_45274398_10000/LConn3 -- T_86014138__/LConn3 -- bus51/LConn1
  _CN_86014138_10000_CN_45274398_10000/RConn1 -- T_45274398__/LConn1 -- _CN_45274398_10000_CN_86204823_10000/LConn1
  _CN_86014138_10000_CN_45274398_10000/RConn2 -- T_45274398__/LConn2 -- _CN_45274398_10000_CN_86204823_10000/LConn2
  _CN_86014138_10000_CN_45274398_10000/RConn3 -- T_45274398__/LConn3 -- _CN_45274398_10000_CN_86204823_10000/LConn3 -- bus52/LConn1
  _CN_92235455_10000_CN_92385756_10000/LConn1 -- T_92235455__/RConn1 -- L_92235455/LConn1
  _CN_92235455_10000_CN_92385756_10000/LConn2 -- T_92235455__/RConn2 -- L_92235455/LConn2
  _CN_92235455_10000_CN_92385756_10000/LConn3 -- T_92235455__/RConn3 -- L_92235455/LConn3 -- bus53/LConn1
  T_92385756__/LConn1 -- _CN_92235455_10000_CN_92385756_10000/RConn1
  T_92385756__/LConn2 -- _CN_92235455_10000_CN_92385756_10000/RConn2
  _CN_92235455_10000_CN_92385756_10000/RConn3 -- T_92385756__/LConn3 -- bus54/LConn1
  T_99501943__/LConn1 -- _CN_99501943_10000_CN_99501945_10000/LConn1
  T_99501943__/LConn2 -- _CN_99501943_10000_CN_99501945_10000/LConn2
  _CN_99501943_10000_CN_99501945_10000/LConn3 -- T_99501943__/LConn3 -- bus55/LConn1
  T_99501945__/LConn1 -- _CN_99501943_10000_CN_99501945_10000/RConn1
  T_99501945__/LConn2 -- _CN_99501943_10000_CN_99501945_10000/RConn2
  _CN_99501943_10000_CN_99501945_10000/RConn3 -- T_99501945__/LConn3 -- bus56/LConn1
  T_86991568__/LConn1 -- _CN_86991568_10000_CN_70241048_10000/LConn1
  T_86991568__/LConn2 -- _CN_86991568_10000_CN_70241048_10000/LConn2
  _CN_86991568_10000_CN_70241048_10000/LConn3 -- T_86991568__/LConn3 -- bus57/LConn1
  T_70241048__/LConn1 -- _CN_86991568_10000_CN_70241048_10000/RConn1
  T_70241048__/LConn2 -- _CN_86991568_10000_CN_70241048_10000/RConn2
  _CN_86991568_10000_CN_70241048_10000/RConn3 -- T_70241048__/LConn3 -- bus58/LConn1
  _CN_117198289_10000_CN_41794316_10000/RConn1 -- T_117198289__/RConn1 -- L_117198289/LConn1
  _CN_117198289_10000_CN_41794316_10000/RConn2 -- T_117198289__/RConn2 -- L_117198289/LConn2
  _CN_117198289_10000_CN_41794316_10000/RConn3 -- T_117198289__/RConn3 -- L_117198289/LConn3 -- bus59/LConn1
  T_86204823__/LConn1 -- _CN_45274398_10000_CN_86204823_10000/RConn1
  T_86204823__/LConn2 -- _CN_45274398_10000_CN_86204823_10000/RConn2
  _CN_45274398_10000_CN_86204823_10000/RConn3 -- T_86204823__/LConn3 -- bus60/LConn1
  "T_33187300__PDC_6_\"Tractoare\""/LConn1 -- _CN_33187294_10000_CN_33187300_10000/RConn1
  "T_33187300__PDC_6_\"Tractoare\""/LConn2 -- _CN_33187294_10000_CN_33187300_10000/RConn2
  _CN_33187294_10000_CN_33187300_10000/RConn3 -- "T_33187300__PDC_6_\"Tractoare\""/LConn3 -- bus61/LConn1
  T_109866037__/LConn1 -- _CN_109866037_10000_CN_50338664_10000/LConn1
  T_109866037__/LConn2 -- _CN_109866037_10000_CN_50338664_10000/LConn2
  _CN_109866037_10000_CN_50338664_10000/LConn3 -- T_109866037__/LConn3 -- bus62/LConn1
  T_50338664__/LConn1 -- _CN_109866037_10000_CN_50338664_10000/RConn1
  T_50338664__/LConn2 -- _CN_109866037_10000_CN_50338664_10000/RConn2
  _CN_109866037_10000_CN_50338664_10000/RConn3 -- T_50338664__/LConn3 -- bus63/LConn1
  T_88266573__/LConn1 -- _CN_88266573_10000_CN_88269277_10000/LConn1
  T_88266573__/LConn2 -- _CN_88266573_10000_CN_88269277_10000/LConn2
  _CN_88266573_10000_CN_88269277_10000/LConn3 -- T_88266573__/LConn3 -- bus64/LConn1
  T_88269277__/LConn1 -- _CN_88266573_10000_CN_88269277_10000/RConn1
  T_88269277__/LConn2 -- _CN_88266573_10000_CN_88269277_10000/RConn2
  _CN_88266573_10000_CN_88269277_10000/RConn3 -- T_88269277__/LConn3 -- bus65/LConn1
  "T_33347441_110000_PDC_28_\"Petricani\""/LConn1 -- _CN_33347441_10000_CN_33309053_10000/LConn1
  "T_33347441_110000_PDC_28_\"Petricani\""/LConn2 -- _CN_33347441_10000_CN_33309053_10000/LConn2
  _CN_33347441_10000_CN_33309053_10000/LConn3 -- "T_33347441_110000_PDC_28_\"Petricani\""/LConn3 -- bus66/LConn1
  "T_33309053__PDC_18_\"Alfa\""/LConn1 -- _CN_33347441_10000_CN_33309053_10000/RConn1
  "T_33309053__PDC_18_\"Alfa\""/LConn2 -- _CN_33347441_10000_CN_33309053_10000/RConn2
  _CN_33347441_10000_CN_33309053_10000/RConn3 -- "T_33309053__PDC_18_\"Alfa\""/LConn3 -- bus67/LConn1
  T_89071477__/LConn1 -- _CN_89071477_10000_CN_46269303_10000/LConn1
  T_89071477__/LConn2 -- _CN_89071477_10000_CN_46269303_10000/LConn2
  _CN_89071477_10000_CN_46269303_10000/LConn3 -- T_89071477__/LConn3 -- bus68/LConn1
  T_46269303__/LConn1 -- _CN_89071477_10000_CN_46269303_10000/RConn1
  T_46269303__/LConn2 -- _CN_89071477_10000_CN_46269303_10000/RConn2
  _CN_89071477_10000_CN_46269303_10000/RConn3 -- T_46269303__/LConn3 -- bus69/LConn1
  T_99475346__/LConn1 -- _CN_99475346_10000_CN_99475378_10000/LConn1
  T_99475346__/LConn2 -- _CN_99475346_10000_CN_99475378_10000/LConn2
  _CN_99475346_10000_CN_99475378_10000/LConn3 -- T_99475346__/LConn3 -- bus70/LConn1
  T_99475378__/LConn1 -- _CN_99475346_10000_CN_99475378_10000/RConn1
  T_99475378__/LConn2 -- _CN_99475346_10000_CN_99475378_10000/RConn2
  _CN_99475346_10000_CN_99475378_10000/RConn3 -- T_99475378__/LConn3 -- bus71/LConn1
  T_95063982__/LConn1 -- _CN_95063982_10000_CN_95064014_10000/LConn1
  T_95063982__/LConn2 -- _CN_95063982_10000_CN_95064014_10000/LConn2
  _CN_95063982_10000_CN_95064014_10000/LConn3 -- T_95063982__/LConn3 -- bus72/LConn1
  T_95064014__/LConn1 -- _CN_95063982_10000_CN_95064014_10000/RConn1
  T_95064014__/LConn2 -- _CN_95063982_10000_CN_95064014_10000/RConn2
  _CN_95063982_10000_CN_95064014_10000/RConn3 -- T_95064014__/LConn3 -- bus73/LConn1
  T_92385772__/LConn1 -- _CN_95423979_10000_CN_92385772_10000/RConn1
  T_92385772__/LConn2 -- _CN_95423979_10000_CN_92385772_10000/RConn2
  _CN_95423979_10000_CN_92385772_10000/RConn3 -- T_92385772__/LConn3 -- bus74/LConn1
  T_56313991__/LConn1 -- _CN_56313991_33000_CN_85644091_33000/LConn1
  T_56313991__/LConn2 -- _CN_56313991_33000_CN_85644091_33000/LConn2
  _CN_56313991_33000_CN_85644091_33000/LConn3 -- T_56313991__/LConn3 -- bus75/LConn1
  T_85644091__/LConn1 -- _CN_56313991_33000_CN_85644091_33000/RConn1
  T_85644091__/LConn2 -- _CN_56313991_33000_CN_85644091_33000/RConn2
  _CN_56313991_33000_CN_85644091_33000/RConn3 -- T_85644091__/LConn3 -- bus76/LConn1
  _CN_27835275_33000_CN_40426094_33000/LConn1 -- "T_27835275__PDC_\"Chișinău_Sud\""/RConn1 -- _CN_27835275_33000_CN_223166735_33000/LConn1
  _CN_27835275_33000_CN_40426094_33000/LConn2 -- "T_27835275__PDC_\"Chișinău_Sud\""/RConn2 -- _CN_27835275_33000_CN_223166735_33000/LConn2
  _CN_27835275_33000_CN_40426094_33000/LConn3 -- "T_27835275__PDC_\"Chișinău_Sud\""/RConn3 -- _CN_27835275_33000_CN_223166735_33000/LConn3 -- bus77/LConn1
  _CN_27835275_33000_CN_40426094_33000/RConn1 -- T_40426094__/LConn1 -- Bălți_Strășeni_CN_41794316_33000_CN_40426094_33000/LConn1
  _CN_27835275_33000_CN_40426094_33000/RConn2 -- T_40426094__/LConn2 -- Bălți_Strășeni_CN_41794316_33000_CN_40426094_33000/LConn2
  _CN_27835275_33000_CN_40426094_33000/RConn3 -- T_40426094__/LConn3 -- Bălți_Strășeni_CN_41794316_33000_CN_40426094_33000/LConn3 -- bus78/LConn1
  T_223166735__/LConn1 -- _CN_27835275_33000_CN_223166735_33000/RConn1
  T_223166735__/LConn2 -- _CN_27835275_33000_CN_223166735_33000/RConn2
  _CN_27835275_33000_CN_223166735_33000/RConn3 -- T_223166735__/LConn3 -- bus79/LConn1
  T_41794316__/LConn1 -- Bălți_Strășeni_CN_41794316_33000_CN_40426094_33000/RConn1
  T_41794316__/LConn2 -- Bălți_Strășeni_CN_41794316_33000_CN_40426094_33000/RConn2
  Bălți_Strășeni_CN_41794316_33000_CN_40426094_33000/RConn3 -- T_41794316__/LConn3 -- bus80/LConn1
  T_49437766__/LConn1 -- _CN_49437766_33000_CN_49437765_33000/LConn1
  T_49437766__/LConn2 -- _CN_49437766_33000_CN_49437765_33000/LConn2
  _CN_49437766_33000_CN_49437765_33000/LConn3 -- T_49437766__/LConn3 -- bus81/LConn1
  T_49437765__/LConn1 -- _CN_49437766_33000_CN_49437765_33000/RConn1
  T_49437765__/LConn2 -- _CN_49437766_33000_CN_49437765_33000/RConn2
  _CN_49437766_33000_CN_49437765_33000/RConn3 -- T_49437765__/LConn3 -- bus82/LConn1
  T_93339994__/LConn1 -- _CN_93339994_33000_CN_81257651_33000/LConn1
  T_93339994__/LConn2 -- _CN_93339994_33000_CN_81257651_33000/LConn2
  _CN_93339994_33000_CN_81257651_33000/LConn3 -- T_93339994__/LConn3 -- bus83/LConn1
  T_81257651__/LConn1 -- _CN_93339994_33000_CN_81257651_33000/RConn1
  T_81257651__/LConn2 -- _CN_93339994_33000_CN_81257651_33000/RConn2
  _CN_93339994_33000_CN_81257651_33000/RConn3 -- T_81257651__/LConn3 -- bus84/LConn1
  _CN_43176990_33000_CN_43201849_33000/LConn1 -- T_43176990__/LConn1 -- _CN_43176990_33000_CN_94086103_33000/LConn1 -- _CN_43176990_33000_CN_43592518_33000/LConn1
  _CN_43176990_33000_CN_43201849_33000/LConn2 -- T_43176990__/LConn2 -- _CN_43176990_33000_CN_94086103_33000/LConn2 -- _CN_43176990_33000_CN_43592518_33000/LConn2
  _CN_43176990_33000_CN_43201849_33000/LConn3 -- T_43176990__/LConn3 -- _CN_43176990_33000_CN_94086103_33000/LConn3 -- _CN_43176990_33000_CN_43592518_33000/LConn3 -- bus85/LConn1
  T_43201849__подстанция_Южная/LConn1 -- _CN_43176990_33000_CN_43201849_33000/RConn1
  T_43201849__подстанция_Южная/LConn2 -- _CN_43176990_33000_CN_43201849_33000/RConn2
  _CN_43176990_33000_CN_43201849_33000/RConn3 -- T_43201849__подстанция_Южная/LConn3 -- bus86/LConn1
  T_94086103__/LConn1 -- _CN_43176990_33000_CN_94086103_33000/RConn1
  T_94086103__/LConn2 -- _CN_43176990_33000_CN_94086103_33000/RConn2
  _CN_43176990_33000_CN_94086103_33000/RConn3 -- T_94086103__/LConn3 -- bus87/LConn1
  T_43592518__/LConn1 -- _CN_43176990_33000_CN_43592518_33000/RConn1
  T_43592518__/LConn2 -- _CN_43176990_33000_CN_43592518_33000/RConn2
  _CN_43176990_33000_CN_43592518_33000/RConn3 -- T_43592518__/LConn3 -- bus88/LConn1
  T_51261349__/LConn1 -- _CN_51261349_33000_CN_57741010_33000/LConn1
  T_51261349__/LConn2 -- _CN_51261349_33000_CN_57741010_33000/LConn2
  _CN_51261349_33000_CN_57741010_33000/LConn3 -- T_51261349__/LConn3 -- bus89/LConn1
  T_57741010__/LConn1 -- _CN_51261349_33000_CN_57741010_33000/RConn1
  T_57741010__/LConn2 -- _CN_51261349_33000_CN_57741010_33000/RConn2
  _CN_51261349_33000_CN_57741010_33000/RConn3 -- T_57741010__/LConn3 -- bus90/LConn1
  T_44112166__/LConn1 -- _CN_44112166_33000_CN_39742580_33000/LConn1
  T_44112166__/LConn2 -- _CN_44112166_33000_CN_39742580_33000/LConn2
  _CN_44112166_33000_CN_39742580_33000/LConn3 -- T_44112166__/LConn3 -- bus91/LConn1
  T_39742580__/LConn1 -- _CN_44112166_33000_CN_39742580_33000/RConn1
  T_39742580__/LConn2 -- _CN_44112166_33000_CN_39742580_33000/RConn2
  _CN_44112166_33000_CN_39742580_33000/RConn3 -- T_39742580__/LConn3 -- bus92/LConn1
  T_49516592__/LConn1 -- _CN_49516592_33000_CN_91215205_33000/LConn1
  T_49516592__/LConn2 -- _CN_49516592_33000_CN_91215205_33000/LConn2
  _CN_49516592_33000_CN_91215205_33000/LConn3 -- T_49516592__/LConn3 -- bus93/LConn1
  T_91215205__/LConn1 -- _CN_49516592_33000_CN_91215205_33000/RConn1
  T_91215205__/LConn2 -- _CN_49516592_33000_CN_91215205_33000/RConn2
  _CN_49516592_33000_CN_91215205_33000/RConn3 -- T_91215205__/LConn3 -- bus94/LConn1
  T_85256767__/LConn1 -- _CN_85256767_33000_CN_92235455_33000/LConn1
  T_85256767__/LConn2 -- _CN_85256767_33000_CN_92235455_33000/LConn2
  _CN_85256767_33000_CN_92235455_33000/LConn3 -- T_85256767__/LConn3 -- bus95/LConn1
  T_92235455__/LConn1 -- _CN_85256767_33000_CN_92235455_33000/RConn1
  T_92235455__/LConn2 -- _CN_85256767_33000_CN_92235455_33000/RConn2
  _CN_85256767_33000_CN_92235455_33000/RConn3 -- T_92235455__/LConn3 -- bus96/LConn1
  T_92224085__/LConn1 -- _CN_92224085_33000_CN_92224090_33000/LConn1
  T_92224085__/LConn2 -- _CN_92224085_33000_CN_92224090_33000/LConn2
  _CN_92224085_33000_CN_92224090_33000/LConn3 -- T_92224085__/LConn3 -- bus97/LConn1
  T_92224090__/LConn1 -- _CN_92224085_33000_CN_92224090_33000/RConn1
  T_92224090__/LConn2 -- _CN_92224085_33000_CN_92224090_33000/RConn2
  _CN_92224085_33000_CN_92224090_33000/RConn3 -- T_92224090__/LConn3 -- bus98/LConn1
  T_46584322__/LConn1 -- _CN_46584322_35000_CN_64202145_35000/LConn1
  T_46584322__/LConn2 -- _CN_46584322_35000_CN_64202145_35000/LConn2
  _CN_46584322_35000_CN_64202145_35000/LConn3 -- T_46584322__/LConn3 -- bus99/LConn1
  T_64202145__/LConn1 -- _CN_46584322_35000_CN_64202145_35000/RConn1
  T_64202145__/LConn2 -- _CN_46584322_35000_CN_64202145_35000/RConn2
  _CN_46584322_35000_CN_64202145_35000/RConn3 -- T_64202145__/LConn3 -- bus100/LConn1
  "T_27835275__PDC_\"Chișinău_Sud\""/LConn1 -- _CN_27835275_35000_CN_47448242_35000/LConn1
  "T_27835275__PDC_\"Chișinău_Sud\""/LConn2 -- _CN_27835275_35000_CN_47448242_35000/LConn2
  _CN_27835275_35000_CN_47448242_35000/LConn3 -- "T_27835275__PDC_\"Chișinău_Sud\""/LConn3 -- bus101/LConn1
  "T_47448242__PDC_36_\"BĂCIOI\""/LConn1 -- _CN_27835275_35000_CN_47448242_35000/RConn1
  "T_47448242__PDC_36_\"BĂCIOI\""/LConn2 -- _CN_27835275_35000_CN_47448242_35000/RConn2
  _CN_27835275_35000_CN_47448242_35000/RConn3 -- "T_47448242__PDC_36_\"BĂCIOI\""/LConn3 -- bus102/LConn1
  T_43840150__/LConn1 -- _CN_43840150_35000_CN_117198289_35000/LConn1
  T_43840150__/LConn2 -- _CN_43840150_35000_CN_117198289_35000/LConn2
  _CN_43840150_35000_CN_117198289_35000/LConn3 -- T_43840150__/LConn3 -- bus103/LConn1
  T_117198289__/LConn1 -- _CN_43840150_35000_CN_117198289_35000/RConn1
  T_117198289__/LConn2 -- _CN_43840150_35000_CN_117198289_35000/RConn2
  _CN_43840150_35000_CN_117198289_35000/RConn3 -- T_117198289__/LConn3 -- bus104/LConn1
  T_43840161__/LConn1 -- _CN_43840161_35000_CN_50226677_35000/LConn1
  T_43840161__/LConn2 -- _CN_43840161_35000_CN_50226677_35000/LConn2
  _CN_43840161_35000_CN_50226677_35000/LConn3 -- T_43840161__/LConn3 -- bus105/LConn1
  T_50226677__/LConn1 -- _CN_43840161_35000_CN_50226677_35000/RConn1
  T_50226677__/LConn2 -- _CN_43840161_35000_CN_50226677_35000/RConn2
  _CN_43840161_35000_CN_50226677_35000/RConn3 -- T_50226677__/LConn3 -- bus106/LConn1
  T_197246155__/LConn1 -- _CN_197246155_35000_CN_51414899_35000/LConn1
  T_197246155__/LConn2 -- _CN_197246155_35000_CN_51414899_35000/LConn2
  _CN_197246155_35000_CN_51414899_35000/LConn3 -- T_197246155__/LConn3 -- bus107/LConn1
  T_51414899__/LConn1 -- _CN_197246155_35000_CN_51414899_35000/RConn1
  T_51414899__/LConn2 -- _CN_197246155_35000_CN_51414899_35000/RConn2
  _CN_197246155_35000_CN_51414899_35000/RConn3 -- T_51414899__/LConn3 -- bus108/LConn1
  T_169701851__/LConn1 -- _CN_169701851_35000_CN_93040737_35000/LConn1
  T_169701851__/LConn2 -- _CN_169701851_35000_CN_93040737_35000/LConn2
  _CN_169701851_35000_CN_93040737_35000/LConn3 -- T_169701851__/LConn3 -- bus109/LConn1
  T_93040737__/LConn1 -- _CN_169701851_35000_CN_93040737_35000/RConn1
  T_93040737__/LConn2 -- _CN_169701851_35000_CN_93040737_35000/RConn2
  _CN_169701851_35000_CN_93040737_35000/RConn3 -- T_93040737__/LConn3 -- bus110/LConn1
  "T_33437413__PDC_43_\"Floreni\""/LConn1 -- _CN_33437413_35000_CN_33437415_35000/LConn1
  "T_33437413__PDC_43_\"Floreni\""/LConn2 -- _CN_33437413_35000_CN_33437415_35000/LConn2
  _CN_33437413_35000_CN_33437415_35000/LConn3 -- "T_33437413__PDC_43_\"Floreni\""/LConn3 -- bus111/LConn1
  "T_33437415__PDC_17_\"Bubiueci\""/LConn1 -- _CN_33437413_35000_CN_33437415_35000/RConn1
  "T_33437415__PDC_17_\"Bubiueci\""/LConn2 -- _CN_33437413_35000_CN_33437415_35000/RConn2
  _CN_33437413_35000_CN_33437415_35000/RConn3 -- "T_33437415__PDC_17_\"Bubiueci\""/LConn3 -- bus112/LConn1
  T_48374400__/RConn1 -- L_48374400/LConn1
  T_48374400__/RConn2 -- L_48374400/LConn2
  L_48374400/LConn3 -- T_48374400__/RConn3 -- bus113/LConn1
  T_85643780__/RConn1 -- L_85643780/LConn1
  T_85643780__/RConn2 -- L_85643780/LConn2
  L_85643780/LConn3 -- T_85643780__/RConn3 -- bus114/LConn1
  T_83892667__/RConn1 -- L_83892667/LConn1
  T_83892667__/RConn2 -- L_83892667/LConn2
  L_83892667/LConn3 -- T_83892667__/RConn3 -- bus115/LConn1
  T_100419275__/RConn1 -- L_100419275/LConn1
  T_100419275__/RConn2 -- L_100419275/LConn2
  L_100419275/LConn3 -- T_100419275__/RConn3 -- bus116/LConn1
  T_67678755__/RConn1 -- L_67678755/LConn1
  T_67678755__/RConn2 -- L_67678755/LConn2
  L_67678755/LConn3 -- T_67678755__/RConn3 -- bus117/LConn1
  T_93799430__/RConn1 -- L_93799430/LConn1
  T_93799430__/RConn2 -- L_93799430/LConn2
  L_93799430/LConn3 -- T_93799430__/RConn3 -- bus118/LConn1
  "T_33533471__PDC_11_\"Zorile\""/RConn1 -- L_33533471/LConn1
  "T_33533471__PDC_11_\"Zorile\""/RConn2 -- L_33533471/LConn2
  L_33533471/LConn3 -- "T_33533471__PDC_11_\"Zorile\""/RConn3 -- bus119/LConn1
  "T_33187294_110000_PDC_1_\"Sculeni\""/RConn1 -- L_33187294/LConn1
  "T_33187294_110000_PDC_1_\"Sculeni\""/RConn2 -- L_33187294/LConn2
  L_33187294/LConn3 -- "T_33187294_110000_PDC_1_\"Sculeni\""/RConn3 -- bus120/LConn1
  T_104961071__/RConn1 -- L_104961071/LConn1
  T_104961071__/RConn2 -- L_104961071/LConn2
  L_104961071/LConn3 -- T_104961071__/RConn3 -- bus121/LConn1
  T_104845142__/RConn1 -- L_104845142/LConn1
  T_104845142__/RConn2 -- L_104845142/LConn2
  L_104845142/LConn3 -- T_104845142__/RConn3 -- bus122/LConn1
  T_43177004__/RConn1 -- L_43177004/LConn1
  T_43177004__/RConn2 -- L_43177004/LConn2
  L_43177004/LConn3 -- T_43177004__/RConn3 -- bus123/LConn1
  T_43177007__/RConn1 -- L_43177007/LConn1
  T_43177007__/RConn2 -- L_43177007/LConn2
  L_43177007/LConn3 -- T_43177007__/RConn3 -- bus124/LConn1
  T_49437741__/RConn1 -- L_49437741/LConn1
  T_49437741__/RConn2 -- L_49437741/LConn2
  L_49437741/LConn3 -- T_49437741__/RConn3 -- bus125/LConn1
  T_49516591__/RConn1 -- L_49516591/LConn1
  T_49516591__/RConn2 -- L_49516591/LConn2
  L_49516591/LConn3 -- T_49516591__/RConn3 -- bus126/LConn1
  T_89214520__/RConn1 -- L_89214520/LConn1
  T_89214520__/RConn2 -- L_89214520/LConn2
  L_89214520/LConn3 -- T_89214520__/RConn3 -- bus127/LConn1
  T_108303571__/RConn1 -- L_108303571/LConn1
  T_108303571__/RConn2 -- L_108303571/LConn2
  L_108303571/LConn3 -- T_108303571__/RConn3 -- bus128/LConn1
  T_92839994__/RConn1 -- L_92839994/LConn1
  T_92839994__/RConn2 -- L_92839994/LConn2
  L_92839994/LConn3 -- T_92839994__/RConn3 -- bus129/LConn1
  T_51199909__/RConn1 -- L_51199909/LConn1
  T_51199909__/RConn2 -- L_51199909/LConn2
  L_51199909/LConn3 -- T_51199909__/RConn3 -- bus130/LConn1
  T_67678785__/RConn1 -- L_67678785/LConn1
  T_67678785__/RConn2 -- L_67678785/LConn2
  L_67678785/LConn3 -- T_67678785__/RConn3 -- bus131/LConn1
  T_53211725__/RConn1 -- L_53211725/LConn1
  T_53211725__/RConn2 -- L_53211725/LConn2
  L_53211725/LConn3 -- T_53211725__/RConn3 -- bus132/LConn1
  "T_38634061__PDC_35_\"Combinatul_de_Carton\""/RConn1 -- L_38634061/LConn1
  "T_38634061__PDC_35_\"Combinatul_de_Carton\""/RConn2 -- L_38634061/LConn2
  L_38634061/LConn3 -- "T_38634061__PDC_35_\"Combinatul_de_Carton\""/RConn3 -- bus133/LConn1
  T_48274938__/RConn1 -- L_48274938/LConn1
  T_48274938__/RConn2 -- L_48274938/LConn2
  L_48274938/LConn3 -- T_48274938__/RConn3 -- bus134/LConn1
  T_96687188__/RConn1 -- L_96687188/LConn1
  T_96687188__/RConn2 -- L_96687188/LConn2
  L_96687188/LConn3 -- T_96687188__/RConn3 -- bus135/LConn1
  T_44046948__/RConn1 -- L_44046948/LConn1
  T_44046948__/RConn2 -- L_44046948/LConn2
  L_44046948/LConn3 -- T_44046948__/RConn3 -- bus136/LConn1
  T_96689384__/RConn1 -- L_96689384/LConn1
  T_96689384__/RConn2 -- L_96689384/LConn2
  L_96689384/LConn3 -- T_96689384__/RConn3 -- bus137/LConn1
  T_92224738__/RConn1 -- L_92224738/LConn1
  T_92224738__/RConn2 -- L_92224738/LConn2
  L_92224738/LConn3 -- T_92224738__/RConn3 -- bus138/LConn1
  T_93805661__/RConn1 -- L_93805661/LConn1
  T_93805661__/RConn2 -- L_93805661/LConn2
  L_93805661/LConn3 -- T_93805661__/RConn3 -- bus139/LConn1
  T_59611290__/RConn1 -- L_59611290/LConn1
  T_59611290__/RConn2 -- L_59611290/LConn2
  L_59611290/LConn3 -- T_59611290__/RConn3 -- bus140/LConn1
  T_33533030__PDC_13_„Albișoara”/RConn1 -- L_33533030/LConn1
  T_33533030__PDC_13_„Albișoara”/RConn2 -- L_33533030/LConn2
  L_33533030/LConn3 -- T_33533030__PDC_13_„Albișoara”/RConn3 -- bus141/LConn1
  "T_33075316__PDC_12_\"Malina_Noua\""/RConn1 -- L_33075316/LConn1
  "T_33075316__PDC_12_\"Malina_Noua\""/RConn2 -- L_33075316/LConn2
  L_33075316/LConn3 -- "T_33075316__PDC_12_\"Malina_Noua\""/RConn3 -- bus142/LConn1
  T_106050843__/RConn1 -- L_106050843/LConn1
  T_106050843__/RConn2 -- L_106050843/LConn2
  L_106050843/LConn3 -- T_106050843__/RConn3 -- bus143/LConn1
  T_106050849__/RConn1 -- L_106050849/LConn1
  T_106050849__/RConn2 -- L_106050849/LConn2
  L_106050849/LConn3 -- T_106050849__/RConn3 -- bus144/LConn1
  T_46587556__/RConn1 -- L_46587556/LConn1
  T_46587556__/RConn2 -- L_46587556/LConn2
  L_46587556/LConn3 -- T_46587556__/RConn3 -- bus145/LConn1
  T_36056921__/RConn1 -- L_36056921/LConn1
  T_36056921__/RConn2 -- L_36056921/LConn2
  L_36056921/LConn3 -- T_36056921__/RConn3 -- bus146/LConn1
  T_50287787__/RConn1 -- L_50287787/LConn1
  T_50287787__/RConn2 -- L_50287787/LConn2
  L_50287787/LConn3 -- T_50287787__/RConn3 -- bus147/LConn1
  T_50287791__/RConn1 -- L_50287791/LConn1
  T_50287791__/RConn2 -- L_50287791/LConn2
  L_50287791/LConn3 -- T_50287791__/RConn3 -- bus148/LConn1
  T_96335020__/RConn1 -- L_96335020/LConn1
  T_96335020__/RConn2 -- L_96335020/LConn2
  L_96335020/LConn3 -- T_96335020__/RConn3 -- bus149/LConn1
  T_96335030__/RConn1 -- L_96335030/LConn1
  T_96335030__/RConn2 -- L_96335030/LConn2
  L_96335030/LConn3 -- T_96335030__/RConn3 -- bus150/LConn1
  T_96335034__/RConn1 -- L_96335034/LConn1
  T_96335034__/RConn2 -- L_96335034/LConn2
  L_96335034/LConn3 -- T_96335034__/RConn3 -- bus151/LConn1
  T_92235449__/RConn1 -- L_92235449/LConn1
  T_92235449__/RConn2 -- L_92235449/LConn2
  L_92235449/LConn3 -- T_92235449__/RConn3 -- bus152/LConn1
  T_95423979__/RConn1 -- L_95423979/LConn1
  T_95423979__/RConn2 -- L_95423979/LConn2
  L_95423979/LConn3 -- T_95423979__/RConn3 -- bus153/LConn1
  T_86014138__/RConn1 -- L_86014138/LConn1
  T_86014138__/RConn2 -- L_86014138/LConn2
  L_86014138/LConn3 -- T_86014138__/RConn3 -- bus154/LConn1
  T_45274398__/RConn1 -- L_45274398/LConn1
  T_45274398__/RConn2 -- L_45274398/LConn2
  L_45274398/LConn3 -- T_45274398__/RConn3 -- bus155/LConn1
  T_92385756__/RConn1 -- L_92385756/LConn1
  T_92385756__/RConn2 -- L_92385756/LConn2
  L_92385756/LConn3 -- T_92385756__/RConn3 -- bus156/LConn1
  T_99501943__/RConn1 -- L_99501943/LConn1
  T_99501943__/RConn2 -- L_99501943/LConn2
  L_99501943/LConn3 -- T_99501943__/RConn3 -- bus157/LConn1
  T_99501945__/RConn1 -- L_99501945/LConn1
  T_99501945__/RConn2 -- L_99501945/LConn2
  L_99501945/LConn3 -- T_99501945__/RConn3 -- bus158/LConn1
  T_86991568__/RConn1 -- L_86991568/LConn1
  T_86991568__/RConn2 -- L_86991568/LConn2
  L_86991568/LConn3 -- T_86991568__/RConn3 -- bus159/LConn1
  T_70241048__/RConn1 -- L_70241048/LConn1
  T_70241048__/RConn2 -- L_70241048/LConn2
  L_70241048/LConn3 -- T_70241048__/RConn3 -- bus160/LConn1
  T_86204823__/RConn1 -- L_86204823/LConn1
  T_86204823__/RConn2 -- L_86204823/LConn2
  L_86204823/LConn3 -- T_86204823__/RConn3 -- bus161/LConn1
  "T_33187300__PDC_6_\"Tractoare\""/RConn1 -- L_33187300/LConn1
  "T_33187300__PDC_6_\"Tractoare\""/RConn2 -- L_33187300/LConn2
  L_33187300/LConn3 -- "T_33187300__PDC_6_\"Tractoare\""/RConn3 -- bus162/LConn1
  T_109866037__/RConn1 -- L_109866037/LConn1
  T_109866037__/RConn2 -- L_109866037/LConn2
  L_109866037/LConn3 -- T_109866037__/RConn3 -- bus163/LConn1
  T_50338664__/RConn1 -- L_50338664/LConn1
  T_50338664__/RConn2 -- L_50338664/LConn2
  L_50338664/LConn3 -- T_50338664__/RConn3 -- bus164/LConn1
  T_88266573__/RConn1 -- L_88266573/LConn1
  T_88266573__/RConn2 -- L_88266573/LConn2
  L_88266573/LConn3 -- T_88266573__/RConn3 -- bus165/LConn1
  T_88269277__/RConn1 -- L_88269277/LConn1
  T_88269277__/RConn2 -- L_88269277/LConn2
  L_88269277/LConn3 -- T_88269277__/RConn3 -- bus166/LConn1
  "T_33347441_110000_PDC_28_\"Petricani\""/RConn1 -- L_33347441/LConn1
  "T_33347441_110000_PDC_28_\"Petricani\""/RConn2 -- L_33347441/LConn2
  L_33347441/LConn3 -- "T_33347441_110000_PDC_28_\"Petricani\""/RConn3 -- bus167/LConn1
  "T_33309053__PDC_18_\"Alfa\""/RConn1 -- L_33309053/LConn1
  "T_33309053__PDC_18_\"Alfa\""/RConn2 -- L_33309053/LConn2
  L_33309053/LConn3 -- "T_33309053__PDC_18_\"Alfa\""/RConn3 -- bus168/LConn1
  T_89071477__/RConn1 -- L_89071477/LConn1
  T_89071477__/RConn2 -- L_89071477/LConn2
  L_89071477/LConn3 -- T_89071477__/RConn3 -- bus169/LConn1
  T_46269303__/RConn1 -- L_46269303/LConn1
  T_46269303__/RConn2 -- L_46269303/LConn2
  L_46269303/LConn3 -- T_46269303__/RConn3 -- bus170/LConn1
  T_99475346__/RConn1 -- L_99475346/LConn1
  T_99475346__/RConn2 -- L_99475346/LConn2
  L_99475346/LConn3 -- T_99475346__/RConn3 -- bus171/LConn1
  T_99475378__/RConn1 -- L_99475378/LConn1
  T_99475378__/RConn2 -- L_99475378/LConn2
  L_99475378/LConn3 -- T_99475378__/RConn3 -- bus172/LConn1
  T_95063982__/RConn1 -- L_95063982/LConn1
  T_95063982__/RConn2 -- L_95063982/LConn2
  L_95063982/LConn3 -- T_95063982__/RConn3 -- bus173/LConn1
  T_95064014__/RConn1 -- L_95064014/LConn1
  T_95064014__/RConn2 -- L_95064014/LConn2
  L_95064014/LConn3 -- T_95064014__/RConn3 -- bus174/LConn1
  T_92385772__/RConn1 -- L_92385772/LConn1
  T_92385772__/RConn2 -- L_92385772/LConn2
  L_92385772/LConn3 -- T_92385772__/RConn3 -- bus175/LConn1
  T_56313991__/RConn1 -- L_56313991/LConn1
  T_56313991__/RConn2 -- L_56313991/LConn2
  L_56313991/LConn3 -- T_56313991__/RConn3 -- bus176/LConn1
  T_85644091__/RConn1 -- L_85644091/LConn1
  T_85644091__/RConn2 -- L_85644091/LConn2
  L_85644091/LConn3 -- T_85644091__/RConn3 -- bus177/LConn1
  T_223166735__/RConn1 -- L_223166735/LConn1
  T_223166735__/RConn2 -- L_223166735/LConn2
  L_223166735/LConn3 -- T_223166735__/RConn3 -- bus178/LConn1
  T_49437766__/RConn1 -- L_49437766/LConn1
  T_49437766__/RConn2 -- L_49437766/LConn2
  L_49437766/LConn3 -- T_49437766__/RConn3 -- bus179/LConn1
  T_49437765__/RConn1 -- L_49437765/LConn1
  T_49437765__/RConn2 -- L_49437765/LConn2
  L_49437765/LConn3 -- T_49437765__/RConn3 -- bus180/LConn1
  T_93339994__/RConn1 -- L_93339994/LConn1
  T_93339994__/RConn2 -- L_93339994/LConn2
  L_93339994/LConn3 -- T_93339994__/RConn3 -- bus181/LConn1
  T_81257651__/RConn1 -- L_81257651/LConn1
  T_81257651__/RConn2 -- L_81257651/LConn2
  L_81257651/LConn3 -- T_81257651__/RConn3 -- bus182/LConn1
  T_94086103__/RConn1 -- L_94086103/LConn1
  T_94086103__/RConn2 -- L_94086103/LConn2
  L_94086103/LConn3 -- T_94086103__/RConn3 -- bus183/LConn1
  T_43592518__/RConn1 -- L_43592518/LConn1
  T_43592518__/RConn2 -- L_43592518/LConn2
  L_43592518/LConn3 -- T_43592518__/RConn3 -- bus184/LConn1
  T_51261349__/RConn1 -- L_51261349/LConn1
  T_51261349__/RConn2 -- L_51261349/LConn2
  L_51261349/LConn3 -- T_51261349__/RConn3 -- bus185/LConn1
  T_57741010__/RConn1 -- L_57741010/LConn1
  T_57741010__/RConn2 -- L_57741010/LConn2
  L_57741010/LConn3 -- T_57741010__/RConn3 -- bus186/LConn1
  T_44112166__/RConn1 -- L_44112166/LConn1
  T_44112166__/RConn2 -- L_44112166/LConn2
  L_44112166/LConn3 -- T_44112166__/RConn3 -- bus187/LConn1
  T_39742580__/RConn1 -- L_39742580/LConn1
  T_39742580__/RConn2 -- L_39742580/LConn2
  L_39742580/LConn3 -- T_39742580__/RConn3 -- bus188/LConn1
  T_49516592__/RConn1 -- L_49516592/LConn1
  T_49516592__/RConn2 -- L_49516592/LConn2
  L_49516592/LConn3 -- T_49516592__/RConn3 -- bus189/LConn1
  T_91215205__/RConn1 -- L_91215205/LConn1
  T_91215205__/RConn2 -- L_91215205/LConn2
  L_91215205/LConn3 -- T_91215205__/RConn3 -- bus190/LConn1
  T_92224090__/RConn1 -- L_92224090/LConn1
  T_92224090__/RConn2 -- L_92224090/LConn2
  L_92224090/LConn3 -- T_92224090__/RConn3 -- bus191/LConn1
  T_64202145__/RConn1 -- L_64202145/LConn1
  T_64202145__/RConn2 -- L_64202145/LConn2
  L_64202145/LConn3 -- T_64202145__/RConn3 -- bus192/LConn1
  "T_47448242__PDC_36_\"BĂCIOI\""/RConn1 -- L_47448242/LConn1
  "T_47448242__PDC_36_\"BĂCIOI\""/RConn2 -- L_47448242/LConn2
  L_47448242/LConn3 -- "T_47448242__PDC_36_\"BĂCIOI\""/RConn3 -- bus193/LConn1
  T_43840150__/RConn1 -- L_43840150/LConn1
  T_43840150__/RConn2 -- L_43840150/LConn2
  L_43840150/LConn3 -- T_43840150__/RConn3 -- bus194/LConn1
  T_43840161__/RConn1 -- L_43840161/LConn1
  T_43840161__/RConn2 -- L_43840161/LConn2
  L_43840161/LConn3 -- T_43840161__/RConn3 -- bus195/LConn1
  T_50226677__/RConn1 -- L_50226677/LConn1
  T_50226677__/RConn2 -- L_50226677/LConn2
  L_50226677/LConn3 -- T_50226677__/RConn3 -- bus196/LConn1
  T_197246155__/RConn1 -- L_197246155/LConn1
  T_197246155__/RConn2 -- L_197246155/LConn2
  L_197246155/LConn3 -- T_197246155__/RConn3 -- bus197/LConn1
  T_51414899__/RConn1 -- L_51414899/LConn1
  T_51414899__/RConn2 -- L_51414899/LConn2
  L_51414899/LConn3 -- T_51414899__/RConn3 -- bus198/LConn1
  T_169701851__/RConn1 -- L_169701851/LConn1
  T_169701851__/RConn2 -- L_169701851/LConn2
  L_169701851/LConn3 -- T_169701851__/RConn3 -- bus199/LConn1
  T_93040737__/RConn1 -- L_93040737/LConn1
  T_93040737__/RConn2 -- L_93040737/LConn2
  L_93040737/LConn3 -- T_93040737__/RConn3 -- bus200/LConn1
  "T_33437413__PDC_43_\"Floreni\""/RConn1 -- L_33437413/LConn1
  "T_33437413__PDC_43_\"Floreni\""/RConn2 -- L_33437413/LConn2
  L_33437413/LConn3 -- "T_33437413__PDC_43_\"Floreni\""/RConn3 -- bus201/LConn1
  "T_33437415__PDC_17_\"Bubiueci\""/RConn1 -- L_33437415/LConn1
  "T_33437415__PDC_17_\"Bubiueci\""/RConn2 -- L_33437415/LConn2
  L_33437415/LConn3 -- "T_33437415__PDC_17_\"Bubiueci\""/RConn3 -- bus202/LConn1
